simulink model "masaresorteamoriguadorpato"  (R2018a)
settings: Solver=ode5  StartTime=0.0  StopTime=10.0  RelTol=1e-3  EnableMultiTasking=on
settings Model: Creator=Daniel  LastModifiedBy=Dell
settings DataIOCC: LimitDataPoints=on  SaveFormat=Array
settings OptimizationCC: LifeSpan=inf
settings DebuggingCC: UnderspecifiedInitializationDetection=Classic  MergeDetectMultiDrivingBlocksExec=none  SolverPrmCheckMsg=warning  StateNameClashWarn=warning  SFUnexpectedBacktrackingDiag=warning  SFNoUnconditionalDefaultTransitionDiag=warning  SFExecutionAtInitializationDiag=none
settings HardwareCC: ProdBitPerPointer=32  ProdBitPerSizeT=32  ProdBitPerPtrDiffT=32  ProdLargestAtomicFloat=None  ProdIntDivRoundTo=Undefined  ProdEndianess=Unspecified  ProdWordSize=32  ProdHWDeviceType=32-bit Generic
settings ModelReferenceCC: PropagateSignalLabelsOutOfModel=off
settings CodeAppCC: StateflowObjectComments=on
settings GRTTargetCC: TargetLangStandard=C89/C90 (ANSI)  GeneratePreprocessorConditionals=Disable all
settings ConfigComp: CovMetricSettings=dw  CovHtmlReporting=on  CovSaveCumulativeToWorkspaceVar=on  CovSaveSingleToWorkspaceVar=on  CovExternalEMLEnable=off

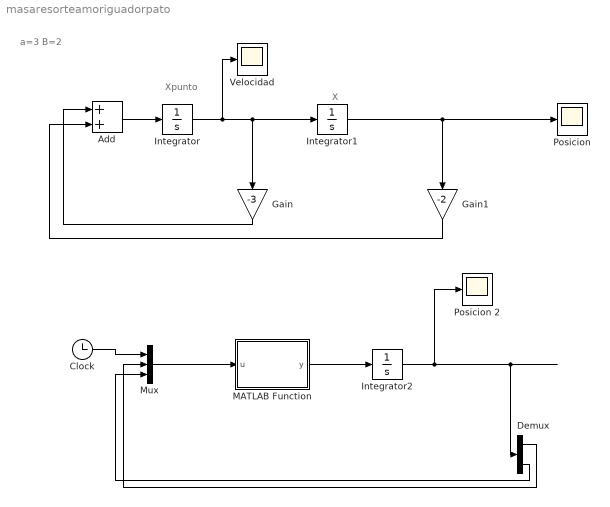
== system masaresorteamoriguadorpato ==
  note: X
  note: Xpunto
  note: a=3
      | B=2
  Add : Sum
  Clock : Clock
  Demux : Demux  Outputs=2
  Gain : Gain  Gain=-3
  Gain1 : Gain  Gain=-2
  Integrator : Integrator  InitialCondition=.1
  Integrator1 : Integrator  InitialCondition=0.3
  Integrator2 : Integrator  InitialCondition=.1
  MATLAB Function : MATLAB Function  TreatAsAtomicUnit=on
  Mux : Mux  Inputs=3
  "Posicion " : Scope
  Posicion 2 : Scope
  Velocidad : Scope
  wires:
  Integrator/1 -> Velocidad/1, Gain/1, Integrator1/1
  Add/1 -> Integrator/1
  Integrator1/1 -> "Posicion "/1, Gain1/1
  Gain/1 -> Add/1
  Gain1/1 -> Add/2
  MATLAB Function/1(y) -> Integrator2/1
  Integrator2/1 -> Demux/1, Posicion 2/1
  Mux/1 -> MATLAB Function/1(u)
  Clock/1 -> Mux/1
  Demux/1 -> Mux/2
  Demux/2 -> Mux/3

== matlab function masaresorteamoriguadorpato/MATLAB Function ==
  data: u input; y output
function y = fcn(u)
u1=u(1);
x1=u(2);
x2=u(3);

dx1=x2;
dx2=(1/6)*(u1-8*x2-2*x1);
y = [dx1,dx2];
